simulink model "Ex3"  (R2017a)
settings: Solver=ode23  StartTime=0.0  StopTime=10.0  RelTol=1e-3  EnableMultiTasking=on
values from neighbouring files (symbols this model uses):
  Jr = 0.746    [ex3Parameters.m]
  Kt = 69.7e-3    (= 0.0697)    [ex3Parameters.m]
libraries: fl_lib x10, nesl_utility x6, simulink x1, elec_lib x1
settings Model: Creator=99641  LastModifiedBy=99641
settings SolverCC: ZeroCrossAlgorithm=Adaptive
settings DataIOCC: LimitDataPoints=on  SaveFormat=Array
settings OptimizationCC: LifeSpan=inf
settings DebuggingCC: SolverPrmCheckMsg=warning  SFUnexpectedBacktrackingDiag=warning  SFNoUnconditionalDefaultTransitionDiag=warning  SFExecutionAtInitializationDiag=none
settings HardwareCC: ProdBitPerPointer=32  ProdBitPerSizeT=32  ProdBitPerPtrDiffT=32  ProdLargestAtomicFloat=None  ProdIntDivRoundTo=Undefined  ProdEndianess=Unspecified  ProdWordSize=32  ProdHWDeviceType=32-bit Generic
settings ModelReferenceCC: PropagateSignalLabelsOutOfModel=off
settings GRTTargetCC: TargetLangStandard=C89/C90 (ANSI)  GeneratePreprocessorConditionals=Disable all
settings ConfigComp: CovMetricSettings=dw  CovHtmlReporting=on  CovSaveCumulativeToWorkspaceVar=on  CovSaveSingleToWorkspaceVar=on  CovExternalEMLEnable=off  CovSFcnEnable=off

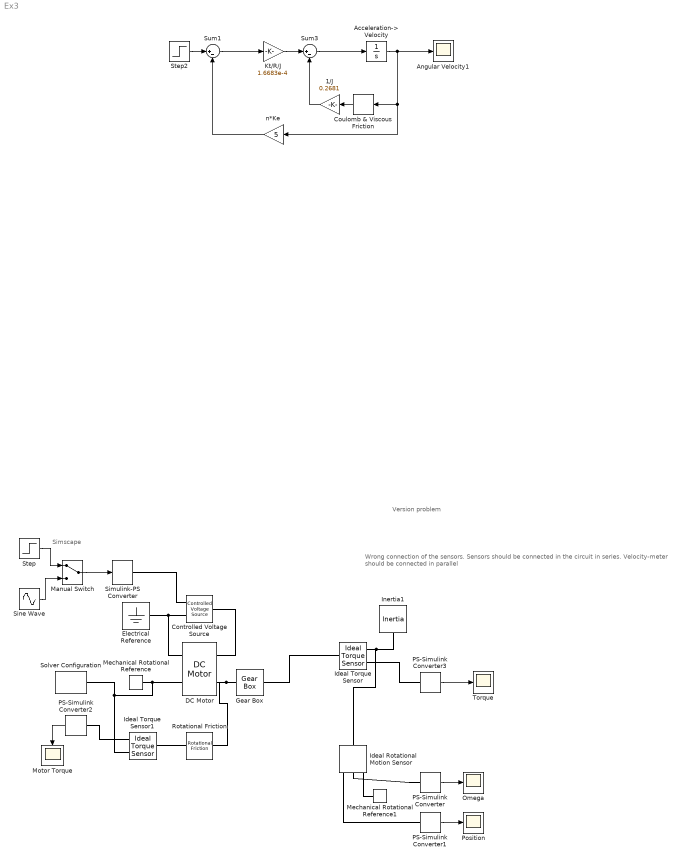
== system Ex3 ==
  note: Version problem
  note: Wrong connection of the sensors.
      | Sensors should be connected in the circuit in series.
      | Velocity-meter should be connected in parallel
  note: Simscape
  " Torque" : Scope
  1/J : Gain  Gain=0.2681
  Acceleration-> Velocity : Integrator
  Angular Velocity1 : Scope
  Controlled Voltage Source : fl_lib/Electrical/Electrical Sources/Controlled Voltage Source
  Coulomb & Viscous Friction : simulink/Discontinuities/Coulomb & Viscous Friction  offset=1e-3  gain=1
      settings: SourceProductName=Simulink
  DC Motor : elec_lib/Actuators & Drivers/Rotational Actuators/DC Motor  parameterization=1  Ra=R Ohm  La=L mH  emf_or_torque=2  Kv=7.2e-5 V/rpm  Ki=Kt N*m/A  T_stall=29.9 N*m  w_max=6440 rpm  w_rated=1.5e+4 rpm  P_rated=0.08 W  V_rated=48 V  J=Jr g*cm^2  lam_param=1  lam=dm N*m/(rad/s)  i_noload=9 mA  V_i_noload=48 V  speed0=0 rpm  alpha=0.00393 1/K  Tmeas=25 C  thermal_mass=100 J/K  initial_temperature=25 C
  Electrical Reference : fl_lib/Electrical/Electrical Elements/Electrical Reference
  Gear Box : fl_lib/Mechanical/Mechanisms/Gear Box  ratio=5  t_in_specify=off  t_in_priority=High  t_in=0 N*m  t_in_nominal_specify=off  t_in_nominal_unit=N*m  t_in_nominal_value=1  t_out_specify=off  t_out_priority=High  t_out=0 N*m  t_out_nominal_specify=off  t_out_nominal_unit=N*m  t_out_nominal_value=1
  Ideal Rotational Motion Sensor : fl_lib/Mechanical/Mechanical Sensors/Ideal Rotational Motion Sensor  offset=0 rad
  Ideal Torque Sensor : fl_lib/Mechanical/Mechanical Sensors/Ideal Torque Sensor
  Ideal Torque Sensor1 : fl_lib/Mechanical/Mechanical Sensors/Ideal Torque Sensor
  Inertia1 : fl_lib/Mechanical/Rotational Elements/Inertia  inertia=Jl kg*m^2  w_specify=off  w_priority=High  w=0 rad/s  w_nominal_specify=off  w_nominal_unit=rad/s  w_nominal_value=1  t_specify=off  t_priority=High  t=0 N*m  t_nominal_specify=off  t_nominal_unit=N*m  t_nominal_value=1
  Kt/R/J : Gain  Gain=1.6683e-4
  Manual Switch : ManualSwitch
  Mechanical Rotational Reference : fl_lib/Mechanical/Rotational Elements/Mechanical Rotational Reference
  Mechanical Rotational Reference1 : fl_lib/Mechanical/Rotational Elements/Mechanical Rotational Reference
  Motor Torque : Scope
  Omega : Scope
  PS-Simulink Converter{,1..3} (4 alike) : nesl_utility/PS-Simulink Converter  PhysicalDomain=network_engine_domain  SubClassName=ps_output  LeftPortType=input  RightPortType=output  PseudoPeriodic=off  Frequencies=[]  Unit=1  AffineConversion=off
  Position : Scope
  Rotational Friction : fl_lib/Mechanical/Rotational Elements/Rotational Friction  brkwy_trq=0.001 N*m  brkwy_vel=0.01 rad/s  Col_trq=0.001 N*m  visc_coef=0 N*m/(rad/s)  w_specify=off  w_priority=High  w=0 rad/s  w_nominal_specify=off  w_nominal_unit=rad/s  w_nominal_value=1  t_specify=off  t_priority=High  t=0 N*m  t_nominal_specify=off  t_nominal_unit=N*m  t_nominal_value=1
      settings: SourceProductName=Simscape
  Simulink-PS Converter : nesl_utility/Simulink-PS Converter  PhysicalDomain=network_engine_domain  SubClassName=ps_input  LeftPortType=input  RightPortType=output  PseudoPeriodic=off  Frequencies=[]  NoiseDistribution=none  NoiseParameters=[]  Unit=1  AffineConversion=off  FilteringAndDerivatives=zero  SimscapeFilterOrder=1  InputFilterTimeConstant=0.001  UdotUserProvided=1
  Sine Wave : Sin  Amplitude=5  SampleTime=0
  Solver Configuration : nesl_utility/Solver Configuration  PhysicalDomain=network_engine_domain  SubClassName=solver  LeftPortType=input  RightPortType=generic  Accelerate=off  Tones=[]  Harmonics=[]  SimulateNoise=off  Profile=off  UseLocalSampling=off  EnableSwitchedLinearOptims=on  FrequencyDomain=off  UseCCode=off  RelTol=0.001  AbsTol=1e-06  MinStep=1e-09  ToWorkspace=off  RevertToSquareIcSolve=off  NumHomotopyIterations=100  PhasorMode=off  PhasorModeNumHarmonics=1  OverrideAbsTol=off  DoDC=off  ResidualTolerance=1e-09  UseLocalSolver=on  LocalSolverChoice=NE_TRAPEZOIDAL_ADVANCER  LocalSolverSampleTime=0.001  DoFixedCost=on  MaxNonlinIter=3  MaxModeIter=2  LinearAlgebra=Sparse  DelaysMemoryBudget=1024  AutomaticFiltering=on  FilteringTimeConstant=0.001
  Step : Step  After=20  SampleTime=0
  Step2 : Step  SampleTime=0
  Sum1 : Sum  Inputs=|+-
  Sum3 : Sum  Inputs=|+-
  n*Ke : Gain  Gain=5
  wires:
  PS-Simulink Converter/1 -> Omega/1
  PS-Simulink Converter1/1 -> Position/1
  PS-Simulink Converter2/1 -> Motor Torque/1
  PS-Simulink Converter3/1 -> " Torque"/1
  Sum3/1 -> Acceleration-> Velocity/1
  Acceleration-> Velocity/1 -> Angular Velocity1/1, Coulomb & Viscous Friction/1, n*Ke/1
  Sum1/1 -> Kt/R/J/1
  Kt/R/J/1 -> Sum3/1
  n*Ke/1 -> Sum1/2
  Step2/1 -> Sum1/1
  Coulomb & Viscous Friction/1 -> 1/J/1
  1/J/1 -> Sum3/2
  Step/1 -> Manual Switch/1
  Sine Wave/1 -> Manual Switch/2
  Manual Switch/1 -> Simulink-PS Converter/1
  connections:
  Mechanical Rotational Reference/LConn1 -- Solver Configuration/RConn1 -- Ideal Torque Sensor1/RConn1 -- DC Motor/RConn2
  Ideal Rotational Motion Sensor/RConn3 -- PS-Simulink Converter1/LConn1
  Controlled Voltage Source/LConn1 -- DC Motor/LConn1
  PS-Simulink Converter/LConn1 -- Ideal Rotational Motion Sensor/RConn2
  Gear Box/LConn1 -- Rotational Friction/RConn1 -- DC Motor/LConn2
  Electrical Reference/LConn1 -- Controlled Voltage Source/RConn2 -- DC Motor/RConn1
  PS-Simulink Converter2/LConn1 -- Ideal Torque Sensor1/RConn2
  Ideal Torque Sensor/RConn2 -- PS-Simulink Converter3/LConn1
  Simulink-PS Converter/RConn1 -- Controlled Voltage Source/RConn1
  Ideal Rotational Motion Sensor/LConn1 -- Inertia1/LConn1 -- Ideal Torque Sensor/RConn1
  Ideal Torque Sensor1/LConn1 -- Rotational Friction/LConn1
  Ideal Torque Sensor/LConn1 -- Gear Box/RConn1
  Mechanical Rotational Reference1/LConn1 -- Ideal Rotational Motion Sensor/RConn1
